simulink model "QuadcopterSimModel_INDI_simple_Atti"  (R2018b)
settings: Solver=ode23  StartTime=0.0  StopTime=1000  FixedStep=sample_time  RelTol=1e-4  EnableMultiTasking=on
undefined symbols (not defined in the file): alt_ground, atmosphere, DiscIntNeverNeededParam, envir, fm_atti, g, jystck, pacer, pos_ref, sigbuilder_block, wind
libraries: unit_conversions_lib x3, aerolibfltsims x2, fmCopterAttiRedIndi_lib x1, filters_lib x1, atmosphere_lib x1, quadcopter_lib x1, aerolibanimutils x1, simulink x1, flightgear_visualization_lib x1, axes_transformation_lib x1, joystick_lib x1
settings Model: Creator=Yannic  LastModifiedBy=yannic
settings SolverCC: ZeroCrossControl=DisableAll
settings DataIOCC: LimitDataPoints=on  ReturnWorkspaceOutputs=on
settings OptimizationCC: LifeSpan=inf
settings DebuggingCC: ReadBeforeWriteMsg=DisableAll  WriteAfterWriteMsg=DisableAll  WriteAfterReadMsg=DisableAll  MultiTaskDSMMsg=none  AllowSymbolicDim=off  LibraryContextMissingDiagnostic=none  SFUnexpectedBacktrackingDiag=warning  SFNoUnconditionalDefaultTransitionDiag=warning  SFExecutionAtInitializationDiag=none
settings ModelReferenceCC: UpdateModelReferenceTargets=IfOutOfDate  PropagateSignalLabelsOutOfModel=off
settings SFSimCC: SFSimEcho=off  SimUseLocalCustomCode=off
settings RTWCC: RTWUseLocalCustomCode=off
settings CodeAppCC: StateflowObjectComments=on
settings GRTTargetCC: TargetLangStandard=C89/C90 (ANSI)
settings ConfigComp: CovMetricSettings=dw  CovHtmlReporting=on  CovSaveCumulativeToWorkspaceVar=on  CovSaveSingleToWorkspaceVar=on  CovExternalEMLEnable=off

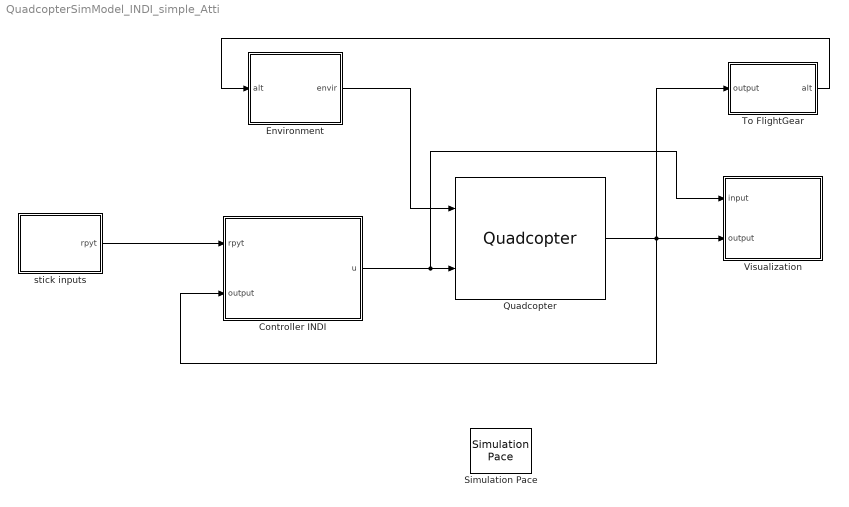
== system QuadcopterSimModel_INDI_simple_Atti ==
  Controller INDI : Subsystem
  Environment : Subsystem
  Quadcopter : quadcopter_lib/Quadcopter  copter_=copter  IC_=IC  grnd_=grnd
      settings: SourceProductName=LADAC
  Simulation Pace : aerolibanimutils/Simulation Pace  SimulationPace=pacer.pace  SleepMode=Auto  OutputPaceError=off  SampleTime=pacer.sample_time
  To FlightGear : Subsystem
  Visualization : Subsystem
  stick inputs : Subsystem
  wires:
  Environment/1(envir) -> Quadcopter/1
  stick inputs/1(rpyt) -> Controller INDI/1(rpyt)
  Quadcopter/1 -> To FlightGear/1(output), Visualization/2(output), Controller INDI/2(output)
  To FlightGear/1(alt) -> Environment/1(alt)
  Controller INDI/1(u) -> Quadcopter/2, Visualization/1(input)

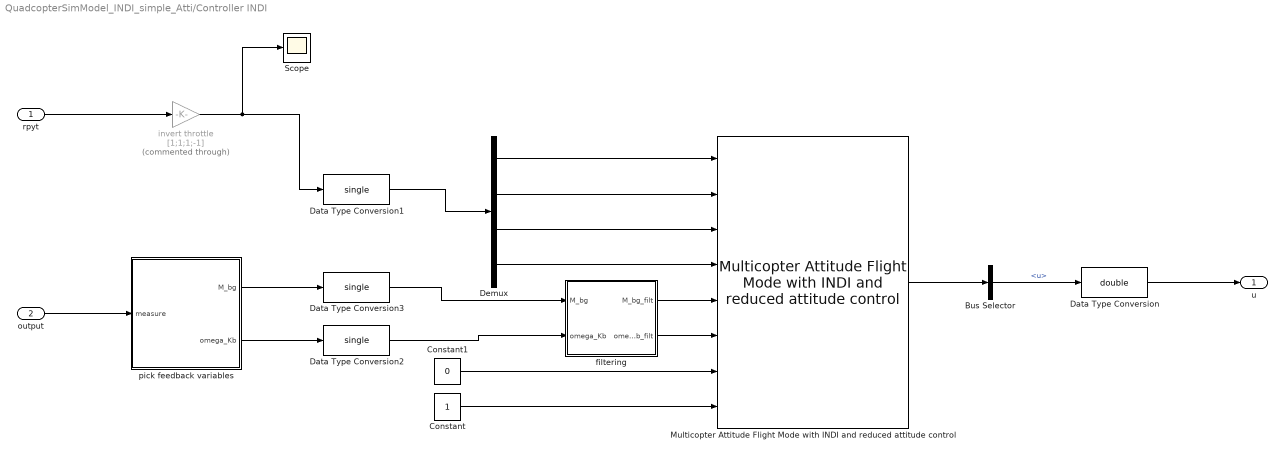
== system QuadcopterSimModel_INDI_simple_Atti/Controller INDI ==
  rpyt : Inport  OutDataTypeStr=double
  output : Inport  Port=2
  Bus Selector : BusSelector  OutputSignals=u
  Constant : Constant  OutDataTypeStr=Inherit: Inherit via back propagation
  Constant1 : Constant  Value=0  OutDataTypeStr=Inherit: Inherit via back propagation
  Data Type Conversion : DataTypeConversion  OutDataTypeStr=double
  Data Type Conversion1 : DataTypeConversion  OutDataTypeStr=single
  Data Type Conversion2 : DataTypeConversion  OutDataTypeStr=single
  Data Type Conversion3 : DataTypeConversion  OutDataTypeStr=single
  Demux : Demux
  Multicopter Attitude Flight Mode with INDI and reduced attitude control : fmCopterAttiRedIndi_lib/Multicopter Attitude Flight Mode with INDI and reduced attitude control  fm=fm_atti
  Scope : Scope
  filtering : Subsystem
  invert throttle : Gain  Commented=through  Gain=[1;1;1;-1]
  pick feedback variables : Subsystem
  u : Outport  OutDataTypeStr=double  PortDimensions=4  SampleTime=[0.0025000000000000001,0]
  wires:
  rpyt/1 -> invert throttle/1
  output/1 -> pick feedback variables/1(measure)
  invert throttle/1 -> Scope/1, Data Type Conversion1/1
  pick feedback variables/2(omega_Kb) -> Data Type Conversion2/1
  pick feedback variables/1(M_bg) -> Data Type Conversion3/1
  Multicopter Attitude Flight Mode with INDI and reduced attitude control/1 -> Bus Selector/1
  Data Type Conversion/1 -> u/1
  Data Type Conversion1/1 -> Demux/1
  Demux/4 -> Multicopter Attitude Flight Mode with INDI and reduced attitude control/4
  Demux/3 -> Multicopter Attitude Flight Mode with INDI and reduced attitude control/3
  Demux/2 -> Multicopter Attitude Flight Mode with INDI and reduced attitude control/2
  Demux/1 -> Multicopter Attitude Flight Mode with INDI and reduced attitude control/1
  Constant/1 -> Multicopter Attitude Flight Mode with INDI and reduced attitude control/8
  Constant1/1 -> Multicopter Attitude Flight Mode with INDI and reduced attitude control/7
  Bus Selector/1 -> Data Type Conversion/1  "<u>"
  Data Type Conversion3/1 -> filtering/1(M_bg)
  filtering/1(M_bg_filt) -> Multicopter Attitude Flight Mode with INDI and reduced attitude control/5
  filtering/2(omega_Kb_filt) -> Multicopter Attitude Flight Mode with INDI and reduced attitude control/6
  Data Type Conversion2/1 -> filtering/2(omega_Kb)

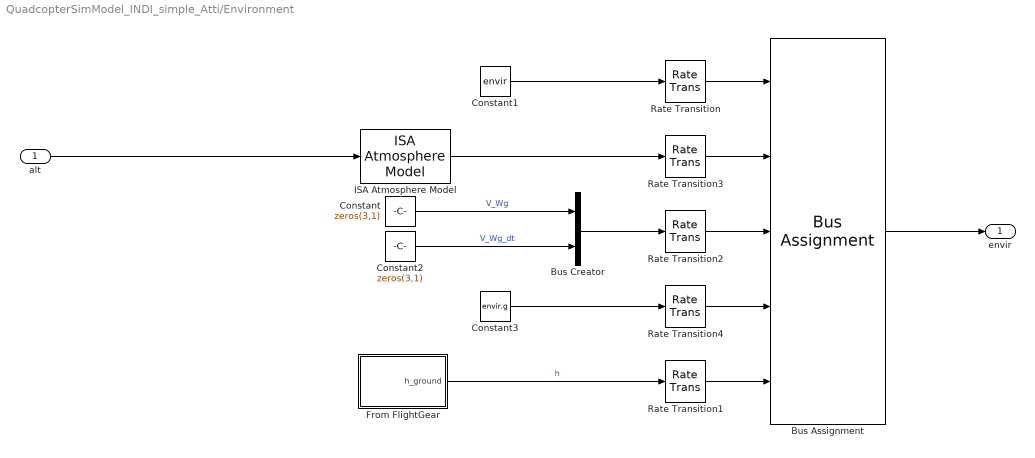
== system QuadcopterSimModel_INDI_simple_Atti/Environment ==
  alt : Inport
  Bus Assignment : BusAssignment  AssignedSignals=atmosphere,wind,g,alt_ground
  Bus Creator : BusCreator  Inputs=2
  Constant : Constant  Value=zeros(3,1)
  Constant1 : Constant  Value=envir  OutDataTypeStr=Bus: envirBus
  Constant2 : Constant  Value=zeros(3,1)
  Constant3 : Constant  Value=envir.g
  From FlightGear : Subsystem
  ISA Atmosphere Model : atmosphere_lib/ISA Atmosphere Model  SystemSampleTime=-1
      settings: SourceProductName=LADAC
  Rate Transition{,1..4} (5 alike) : RateTransition
  envir : Outport
  wires:
  From FlightGear/1(h_ground) -> Rate Transition1/1  "h"
  Rate Transition2/1 -> Bus Assignment/3
  Rate Transition3/1 -> Bus Assignment/2
  Bus Assignment/1 -> envir/1
  Rate Transition/1 -> Bus Assignment/1
  ISA Atmosphere Model/1 -> Rate Transition3/1
  Constant/1 -> Bus Creator/1  "V_Wg"
  Rate Transition1/1 -> Bus Assignment/5
  Constant1/1 -> Rate Transition/1
  alt/1 -> ISA Atmosphere Model/1
  Bus Creator/1 -> Rate Transition2/1
  Constant2/1 -> Bus Creator/2  "V_Wg_dt"
  Rate Transition4/1 -> Bus Assignment/4
  Constant3/1 -> Rate Transition4/1

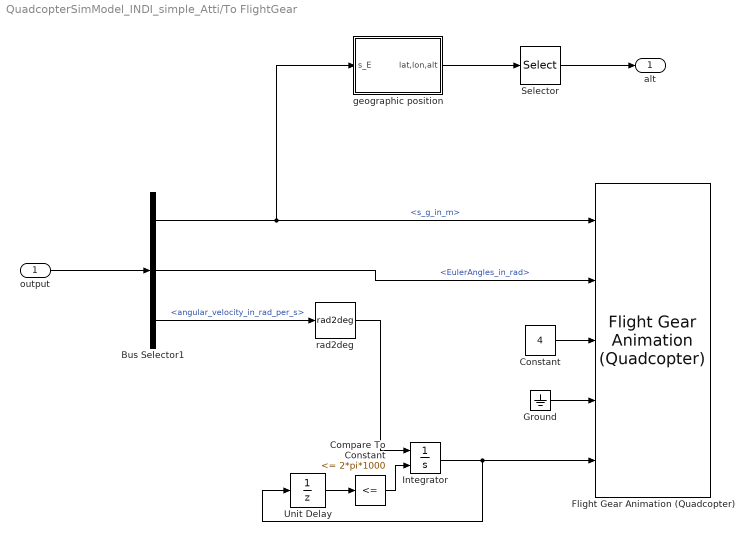
== system QuadcopterSimModel_INDI_simple_Atti/To FlightGear ==
  output : Inport
  Bus Selector1 : BusSelector  OutputSignals=rigidBodyBus.s_g_in_m,rigidBodyBus.EulerAngles_in_rad,motorBus.angular_velocity_in_rad_per_s
  Compare To Constant : simulink/Logic and Bit Operations/Compare To Constant  relop=<=  const=2*pi*1000  OutDataTypeStr=boolean
  Constant : Constant  Value=4
  Flight Gear Animation (Quadcopter) : flightgear_visualization_lib/Flight Gear Animation (Quadcopter)  inital_lat=pos_ref.lat  inital_long=pos_ref.lon  inital_height=pos_ref.alt  remoteURL=fg.remoteURL  remotePort=fg.remotePort
      settings: SourceProductName=LADAC
  Ground : Ground
  Integrator : Integrator  ExternalReset=rising
  Selector : Selector  InputPortWidth=3  IndexOptions=Index vector (dialog)  Indices=3  OutputSizes=1
  Unit Delay : UnitDelay  SampleTime=-1
  geographic position : Subsystem
  rad2deg : unit_conversions_lib/rad2deg
      settings: SourceProductName=LADAC
  alt : Outport
  wires:
  Bus Selector1/1 -> geographic position/1(s_E), Flight Gear Animation (Quadcopter)/1  "<s_g_in_m>"
  output/1 -> Bus Selector1/1
  geographic position/1(lat,lon,alt) -> Selector/1
  Bus Selector1/2 -> Flight Gear Animation (Quadcopter)/2  "<EulerAngles_in_rad>"
  Bus Selector1/3 -> rad2deg/1  "<angular_velocity_in_rad_per_s>"
  Selector/1 -> alt/1
  Constant/1 -> Flight Gear Animation (Quadcopter)/3
  Ground/1 -> Flight Gear Animation (Quadcopter)/4
  Integrator/1 -> Unit Delay/1, Flight Gear Animation (Quadcopter)/5
  Unit Delay/1 -> Compare To Constant/1
  Compare To Constant/1 -> Integrator/2
  rad2deg/1 -> Integrator/1

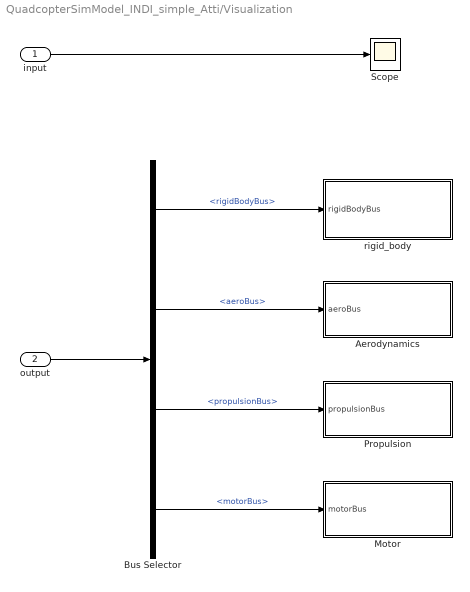
== system QuadcopterSimModel_INDI_simple_Atti/Visualization ==
  input : Inport
  output : Inport  Port=2
  Aerodynamics : Subsystem
  Bus Selector : BusSelector  OutputSignals=rigidBodyBus,aeroBus,propulsionBus,motorBus
  Motor : Subsystem
  Propulsion : Subsystem
  Scope : Scope
  rigid_body : Subsystem
  wires:
  output/1 -> Bus Selector/1
  Bus Selector/1 -> rigid_body/1(rigidBodyBus)  "<rigidBodyBus>"
  Bus Selector/2 -> Aerodynamics/1(aeroBus)  "<aeroBus>"
  Bus Selector/3 -> Propulsion/1(propulsionBus)  "<propulsionBus>"
  Bus Selector/4 -> Motor/1(motorBus)  "<motorBus>"
  input/1 -> Scope/1

== system QuadcopterSimModel_INDI_simple_Atti/stick inputs ==
  Calibrated Joystick : joystick_lib/Calibrated Joystick  jystck=jystck
      settings: SourceProductName=LADAC
  Constant1 : Constant  Value=jystck.enable
  Scope : Scope
  Selector2 : Selector  InputPortWidth=8  IndexOptions=Index vector (dialog)  Indices=[1,2,3,4]  OutputSizes=1
  Signal builder : Subsystem
  Switch1 : Switch  Criteria=u2 > Threshold
  rpyt : Outport
  wires:
  Switch1/1 -> Selector2/1, Scope/1
  Calibrated Joystick/1 -> Switch1/1
  Constant1/1 -> Calibrated Joystick/Enable, Switch1/2
  Signal builder/1(r) -> Switch1/3
  Selector2/1 -> rpyt/1

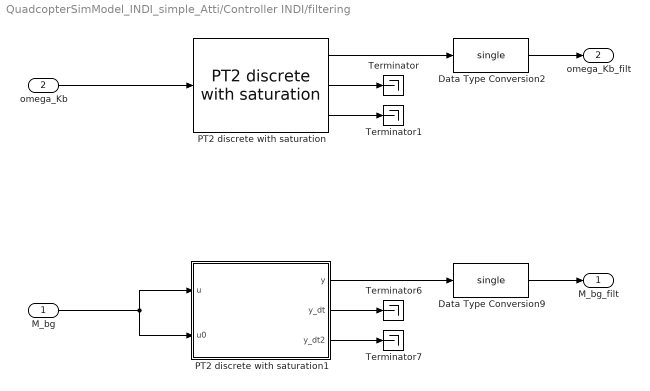
== system QuadcopterSimModel_INDI_simple_Atti/Controller INDI/filtering ==
  M_bg : Inport
  omega_Kb : Inport  Port=2
  Data Type Conversion2 : DataTypeConversion  OutDataTypeStr=single
  Data Type Conversion9 : DataTypeConversion  OutDataTypeStr=single
  PT2 discrete with saturation : filters_lib/PT2 discrete with saturation  omega=fm_atti.sens_filt.omega  d=fm_atti.sens_filt.D  x_dt2_max=inf  x_dt2_min=-inf  x_dt_max=inf  x_dt_min=-inf  x_max=inf  x_min=-inf  x_init=0  x_dt_init=0
      settings: SourceProductName=LADAC
  PT2 discrete with saturation1 : Subsystem  mask{omega=fm_atti.sens_filt.omega, d=fm_atti.sens_filt.D, x_dt2_max=inf, x_dt2_min=-inf, x_dt_max=inf, x_dt_min=-inf, x_max=inf, x_min=-inf, x_init=0, x_dt_init=0}
      mask prompts: omega "Natural frequency"; d "Damping ratio"; x_dt2_max "Maximum acceleration"; x_dt2_min "Minimum acceleration"; x_dt_max "Maximum rate"; x_dt_min "Minimum rate"; x_max "Maximum position"; x_min "Minimum position"; x_init "Initial position"; x_dt_init "Initial rate"
  Terminator{,1,6..7} (4 alike) : Terminator
  M_bg_filt : Outport
  omega_Kb_filt : Outport  Port=2
  wires:
  omega_Kb/1 -> PT2 discrete with saturation/1
  PT2 discrete with saturation/1 -> Data Type Conversion2/1
  M_bg/1 -> PT2 discrete with saturation1/2(u0), PT2 discrete with saturation1/1(u)
  PT2 discrete with saturation1/1(y) -> Data Type Conversion9/1
  PT2 discrete with saturation/2 -> Terminator/1
  PT2 discrete with saturation/3 -> Terminator1/1
  PT2 discrete with saturation1/2(y_dt) -> Terminator6/1
  PT2 discrete with saturation1/3(y_dt2) -> Terminator7/1
  Data Type Conversion9/1 -> M_bg_filt/1
  Data Type Conversion2/1 -> omega_Kb_filt/1

== system QuadcopterSimModel_INDI_simple_Atti/Controller INDI/pick feedback variables ==
  measure : Inport
  Bus Selector1 : BusSelector  OutputSignals=rigidBodyBus.omega_Kb_in_rad_per_s,rigidBodyBus.M_bg_in_1
  M_bg : Outport
  omega_Kb : Outport  Port=2
  wires:
  measure/1 -> Bus Selector1/1
  Bus Selector1/2 -> M_bg/1  "<M_bg_in_1>"
  Bus Selector1/1 -> omega_Kb/1  "<omega_Kb_in_rad_per_s>"

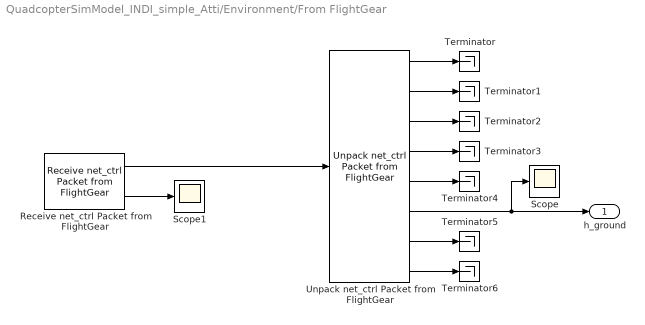
== system QuadcopterSimModel_INDI_simple_Atti/Environment/From FlightGear ==
  Receive net_ctrl Packet from FlightGear : aerolibfltsims/Receive net_ctrl Packet from FlightGear  FlightGearVersion=v3.4  ReceiveAddress=127.0.0.1  ReceivePort=5503  ReceiveWidth=744  varLen=off  SampleTime=1/5  packetFlag=on
      settings: AttributesFormatString=Version Selected:\n%<FlightGearVersion>  SourceProductName=Aerospace Blockset  SourceProductBaseCode=AE
  Scope : Scope
  Scope1 : Scope
  Terminator{,1..6} (7 alike) : Terminator
  Unpack net_ctrl Packet from FlightGear : aerolibfltsims/Unpack net_ctrl Packet from FlightGear  FlightGearVersion=v3.4  ShowControlSurfacePositionOutputs=off  ShowEngineFuelOutputs=off  ShowLandingGearOutputs=off  ShowAvionicOutputs=off  ShowEnvironmentOutputs=on  SampleTime=1/5  packetVersion=27
      settings: AttributesFormatString=Version Selected: %<FlightGearVersion>  SourceProductName=Aerospace Blockset  SourceProductBaseCode=AE
  h_ground : Outport
  wires:
  Unpack net_ctrl Packet from FlightGear/4 -> Terminator3/1
  Unpack net_ctrl Packet from FlightGear/5 -> Terminator4/1
  Receive net_ctrl Packet from FlightGear/1 -> Unpack net_ctrl Packet from FlightGear/1
  Unpack net_ctrl Packet from FlightGear/2 -> Terminator1/1
  Unpack net_ctrl Packet from FlightGear/7 -> Terminator5/1
  Unpack net_ctrl Packet from FlightGear/1 -> Terminator/1
  Unpack net_ctrl Packet from FlightGear/3 -> Terminator2/1
  Unpack net_ctrl Packet from FlightGear/8 -> Terminator6/1
  Unpack net_ctrl Packet from FlightGear/6 -> Scope/1, h_ground/1
  Receive net_ctrl Packet from FlightGear/2 -> Scope1/1

== system QuadcopterSimModel_INDI_simple_Atti/To FlightGear/geographic position ==
  s_E : Inport
  Constant : Constant  Value=pos_ref.lat
  Constant1 : Constant  Value=pos_ref.lon
  Constant2 : Constant  Value=pos_ref.alt
  Mux : Mux  Inputs=3
  Scope : Scope  NumInputPorts=3
  "flat earth to lat, lon, alt" : axes_transformation_lib/NED to lat, lon, alt  SystemSampleTime=-1
      settings: SourceProductName=LADAC
  lat,lon,alt : Outport
  wires:
  Constant2/1 -> "flat earth to lat, lon, alt"/3
  Constant1/1 -> "flat earth to lat, lon, alt"/2
  "flat earth to lat, lon, alt"/3 -> Scope/3, Mux/3
  Constant/1 -> "flat earth to lat, lon, alt"/1
  Mux/1 -> lat,lon,alt/1
  s_E/1 -> "flat earth to lat, lon, alt"/4
  "flat earth to lat, lon, alt"/2 -> Mux/2, Scope/2
  "flat earth to lat, lon, alt"/1 -> Mux/1, Scope/1

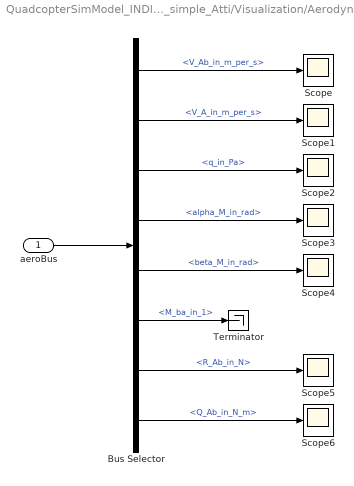
== system QuadcopterSimModel_INDI_simple_Atti/Visualization/Aerodynamics ==
  aeroBus : Inport
  Bus Selector : BusSelector  OutputSignals=V_Ab_in_m_per_s,V_A_in_m_per_s,q_in_Pa,angles.alpha_M_in_rad,angles.beta_M_in_rad,M_ba_in_1,R_Ab_in_N,Q_Ab_in_N_m
  Scope{,1..6} (7 alike) : Scope
  Terminator : Terminator
  wires:
  aeroBus/1 -> Bus Selector/1
  Bus Selector/1 -> Scope/1  "<V_Ab_in_m_per_s>"
  Bus Selector/2 -> Scope1/1  "<V_A_in_m_per_s>"
  Bus Selector/3 -> Scope2/1  "<q_in_Pa>"
  Bus Selector/4 -> Scope3/1  "<alpha_M_in_rad>"
  Bus Selector/5 -> Scope4/1  "<beta_M_in_rad>"
  Bus Selector/6 -> Terminator/1  "<M_ba_in_1>"
  Bus Selector/7 -> Scope5/1  "<R_Ab_in_N>"
  Bus Selector/8 -> Scope6/1  "<Q_Ab_in_N_m>"

== system QuadcopterSimModel_INDI_simple_Atti/Visualization/Motor ==
  motorBus : Inport
  Bus Selector : BusSelector  OutputSignals=angular_acceleration_in_rad_per_square_s,angular_velocity_in_rad_per_s
  Scope : Scope
  Scope1 : Scope
  wires:
  Bus Selector/1 -> Scope/1  "<angular_acceleration_in_rad_per_square_s>"
  motorBus/1 -> Bus Selector/1
  Bus Selector/2 -> Scope1/1  "<angular_velocity_in_rad_per_s>"

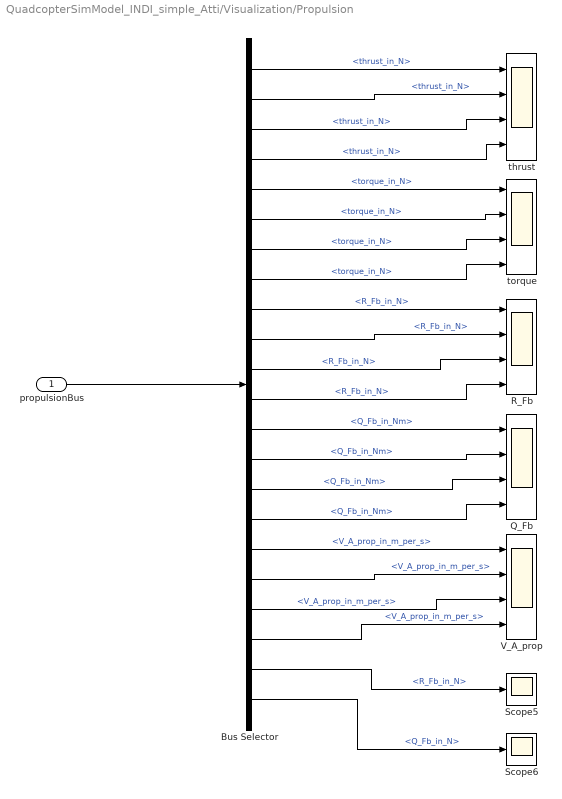
== system QuadcopterSimModel_INDI_simple_Atti/Visualization/Propulsion ==
  propulsionBus : Inport
  Bus Selector : BusSelector  OutputSignals=propeller_1.thrust_in_N,propeller_2.thrust_in_N,propeller_3.thrust_in_N,propeller_4.thrust_in_N,propeller_1.torque_in_N,propeller_2.torque_in_N,propeller_3.torque_in_N,propeller_4.torque_in_N,propeller_1.R_Fb_in_N,propeller_2.R_Fb_in_N,propeller_3.R_Fb_in_N,propeller_4.R_Fb_in_N,propeller_1.Q_Fb_in_Nm,propeller_2.Q_Fb_in_Nm,propeller_3.Q_Fb_in_Nm,propeller_4.Q_Fb_in_Nm,propeller_1.V_A_prop_in_m_per_s,propeller_2.V_A_prop_in_m_per_s,propeller_3.V_A_prop_in_m_per_s,propeller_4.V_A_prop_in_m_per_s,R_Fb_in_N,Q_Fb_in_N
  Q_Fb : Scope  NumInputPorts=4
  R_Fb : Scope  NumInputPorts=4
  Scope5 : Scope
  Scope6 : Scope
  V_A_prop : Scope  NumInputPorts=4
  thrust : Scope  NumInputPorts=4
  torque : Scope  NumInputPorts=4
  wires:
  propulsionBus/1 -> Bus Selector/1
  Bus Selector/1 -> thrust/1  "<thrust_in_N>"
  Bus Selector/2 -> thrust/2  "<thrust_in_N>"
  Bus Selector/3 -> thrust/3  "<thrust_in_N>"
  Bus Selector/4 -> thrust/4  "<thrust_in_N>"
  Bus Selector/5 -> torque/1  "<torque_in_N>"
  Bus Selector/6 -> torque/2  "<torque_in_N>"
  Bus Selector/7 -> torque/3  "<torque_in_N>"
  Bus Selector/8 -> torque/4  "<torque_in_N>"
  Bus Selector/9 -> R_Fb/1  "<R_Fb_in_N>"
  Bus Selector/10 -> R_Fb/2  "<R_Fb_in_N>"
  Bus Selector/11 -> R_Fb/3  "<R_Fb_in_N>"
  Bus Selector/12 -> R_Fb/4  "<R_Fb_in_N>"
  Bus Selector/13 -> Q_Fb/1  "<Q_Fb_in_Nm>"
  Bus Selector/14 -> Q_Fb/2  "<Q_Fb_in_Nm>"
  Bus Selector/15 -> Q_Fb/3  "<Q_Fb_in_Nm>"
  Bus Selector/16 -> Q_Fb/4  "<Q_Fb_in_Nm>"
  Bus Selector/17 -> V_A_prop/1  "<V_A_prop_in_m_per_s>"
  Bus Selector/18 -> V_A_prop/2  "<V_A_prop_in_m_per_s>"
  Bus Selector/19 -> V_A_prop/3  "<V_A_prop_in_m_per_s>"
  Bus Selector/20 -> V_A_prop/4  "<V_A_prop_in_m_per_s>"
  Bus Selector/21 -> Scope5/1  "<R_Fb_in_N>"
  Bus Selector/22 -> Scope6/1  "<Q_Fb_in_N>"

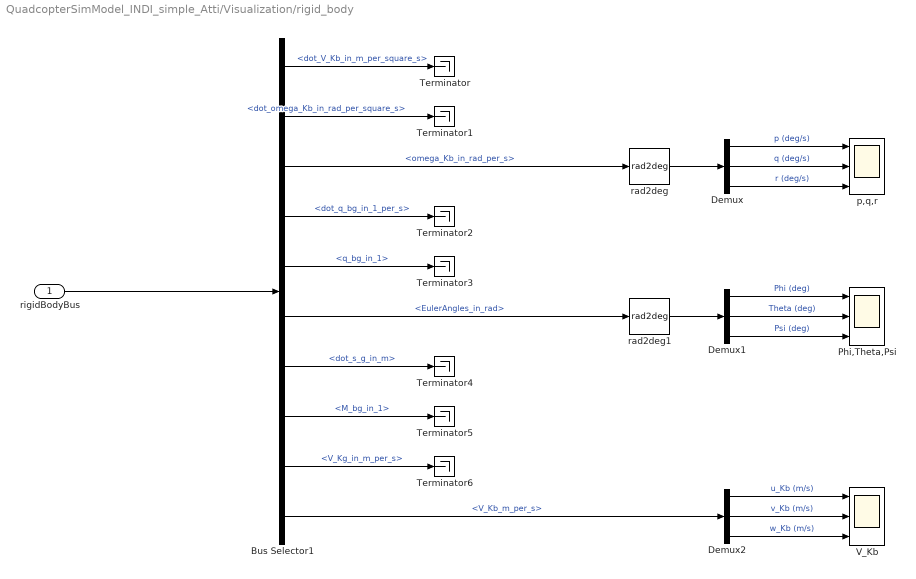
== system QuadcopterSimModel_INDI_simple_Atti/Visualization/rigid_body ==
  rigidBodyBus : Inport
  Bus Selector1 : BusSelector  OutputSignals=dot_V_Kb_in_m_per_square_s,dot_omega_Kb_in_rad_per_square_s,omega_Kb_in_rad_per_s,dot_q_bg_in_1_per_s,q_bg_in_1,EulerAngles_in_rad,dot_s_g_in_m,M_bg_in_1,V_Kg_in_m_per_s,V_Kb_m_per_s
  Demux : Demux  Outputs=3
  Demux1 : Demux  Outputs=3
  Demux2 : Demux  Outputs=3
  Phi,Theta,Psi : Scope  NumInputPorts=3
  Terminator{,1..6} (7 alike) : Terminator
  V_Kb : Scope  NumInputPorts=3
  p,q,r : Scope  NumInputPorts=3
  rad2deg : unit_conversions_lib/rad2deg
      settings: SourceProductName=LADAC
  rad2deg1 : unit_conversions_lib/rad2deg
      settings: SourceProductName=LADAC
  wires:
  Demux/1 -> p,q,r/1  "p (deg/s)"
  Demux1/2 -> Phi,Theta,Psi/2  "Theta (deg)"
  rad2deg/1 -> Demux/1
  Demux1/1 -> Phi,Theta,Psi/1  "Phi (deg)"
  Demux1/3 -> Phi,Theta,Psi/3  "Psi (deg)"
  Demux2/3 -> V_Kb/3  "w_Kb (m/s)"
  Bus Selector1/7 -> Terminator4/1  "<dot_s_g_in_m>"
  Bus Selector1/6 -> rad2deg1/1  "<EulerAngles_in_rad>"
  Bus Selector1/3 -> rad2deg/1  "<omega_Kb_in_rad_per_s>"
  Demux/3 -> p,q,r/3  "r (deg/s)"
  Bus Selector1/1 -> Terminator/1  "<dot_V_Kb_in_m_per_square_s>"
  Demux2/2 -> V_Kb/2  "v_Kb (m/s)"
  Demux/2 -> p,q,r/2  "q (deg/s)"
  rad2deg1/1 -> Demux1/1
  Bus Selector1/5 -> Terminator3/1  "<q_bg_in_1>"
  Demux2/1 -> V_Kb/1  "u_Kb (m/s)"
  Bus Selector1/10 -> Demux2/1  "<V_Kb_m_per_s>"
  rigidBodyBus/1 -> Bus Selector1/1
  Bus Selector1/8 -> Terminator5/1  "<M_bg_in_1>"
  Bus Selector1/4 -> Terminator2/1  "<dot_q_bg_in_1_per_s>"
  Bus Selector1/2 -> Terminator1/1  "<dot_omega_Kb_in_rad_per_square_s>"
  Bus Selector1/9 -> Terminator6/1  "<V_Kg_in_m_per_s>"

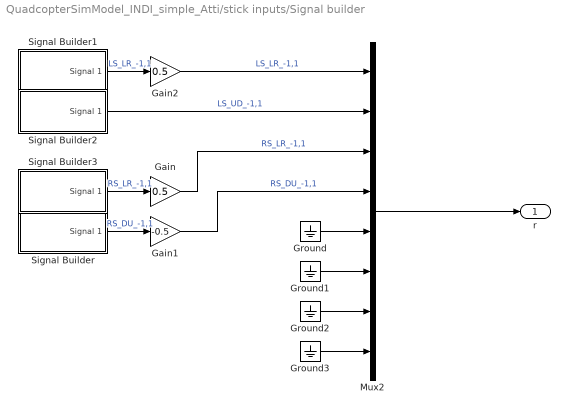
== system QuadcopterSimModel_INDI_simple_Atti/stick inputs/Signal builder ==
  Gain : Gain  Gain=0.5
  Gain1 : Gain  Gain=-0.5
  Gain2 : Gain  Gain=0.5
  Ground{,1..3} (4 alike) : Ground
  Mux2 : Mux  Inputs=8
  Signal Builder : Subsystem  Tag=STV Subsys  LoadFcn=sigbuilder_block('load');  StartFcn=sigbuilder_block('start');  StopFcn=sigbuilder_block('stop');  ClipboardFcn=sigbuilder_block('clipboard');  mask(Sigbuilder block){tuvar=[0:10]}
      mask help: Simulink:masks:SigbuilderBlock_MD
      mask init:
      | if ~strcmp(get_param(bdroot(gcbh),'SimulationStatus'),'stopped') tuvar = sigbuilder_block('maskInit'); end
      settings: CopyFcn=sigbuilder_block('copy');  DeleteFcn=sigbuilder_block('delete');  ModelCloseFcn=sigbuilder_block('modelClose');  PreSaveFcn=sigbuilder_block('preSave');  PauseFcn=sigbuilder_block('pause');  ContinueFcn=sigbuilder_block('continue');  NameChangeFcn=sigbuilder_block('namechange');  OpenFcn=sigbuilder_block('open',[426 42.75 821.25 509.25 ]);  CloseFcn=sigbuilder_block('close');
      mask Display: plot(0, 0, 100, 100,[2, 2, 32, 32, 2], [68, 8, 8, 68, 68],[32, 2], [38, 38], [32, 19, 2],[53, 60, 44], [32, 17, 17, 2],[16, 16, 31, 31]);txt = getActiveGroup(gcbh);text(2, 100, txt,'verticalAlignment', 'top');
  Signal Builder1 : Subsystem  Tag=STV Subsys  LoadFcn=sigbuilder_block('load');  StartFcn=sigbuilder_block('start');  StopFcn=sigbuilder_block('stop');  ClipboardFcn=sigbuilder_block('clipboard');  mask(Sigbuilder block){tuvar=[0:10]}
      mask help: Simulink:masks:SigbuilderBlock_MD
      mask init:
      | if ~strcmp(get_param(bdroot(gcbh),'SimulationStatus'),'stopped') tuvar = sigbuilder_block('maskInit'); end
      settings: CopyFcn=sigbuilder_block('copy');  DeleteFcn=sigbuilder_block('delete');  ModelCloseFcn=sigbuilder_block('modelClose');  PreSaveFcn=sigbuilder_block('preSave');  PauseFcn=sigbuilder_block('pause');  ContinueFcn=sigbuilder_block('continue');  NameChangeFcn=sigbuilder_block('namechange');  OpenFcn=sigbuilder_block('open',[429.75 123 565.5 444.75 ]);  CloseFcn=sigbuilder_block('close');
      mask Display: plot(0, 0, 100, 100,[2, 2, 32, 32, 2], [68, 8, 8, 68, 68],[32, 2], [38, 38], [32, 19, 2],[53, 60, 44], [32, 17, 17, 2],[16, 16, 31, 31]);txt = getActiveGroup(gcbh);text(2, 100, txt,'verticalAlignment', 'top');
  Signal Builder2 : Subsystem  Tag=STV Subsys  LoadFcn=sigbuilder_block('load');  StartFcn=sigbuilder_block('start');  StopFcn=sigbuilder_block('stop');  ClipboardFcn=sigbuilder_block('clipboard');  mask(Sigbuilder block){tuvar=[0:10]}
      mask help: Simulink:masks:SigbuilderBlock_MD
      mask init:
      | if ~strcmp(get_param(bdroot(gcbh),'SimulationStatus'),'stopped') tuvar = sigbuilder_block('maskInit'); end
      settings: CopyFcn=sigbuilder_block('copy');  DeleteFcn=sigbuilder_block('delete');  ModelCloseFcn=sigbuilder_block('modelClose');  PreSaveFcn=sigbuilder_block('preSave');  PauseFcn=sigbuilder_block('pause');  ContinueFcn=sigbuilder_block('continue');  NameChangeFcn=sigbuilder_block('namechange');  OpenFcn=sigbuilder_block('open',[411 0 603 557.25 ]);  CloseFcn=sigbuilder_block('close');
      mask Display: plot(0, 0, 100, 100,[2, 2, 32, 32, 2], [68, 8, 8, 68, 68],[32, 2], [38, 38], [32, 19, 2],[53, 60, 44], [32, 17, 17, 2],[16, 16, 31, 31]);txt = getActiveGroup(gcbh);text(2, 100, txt,'verticalAlignment', 'top');
  Signal Builder3 : Subsystem  Tag=STV Subsys  LoadFcn=sigbuilder_block('load');  StartFcn=sigbuilder_block('start');  StopFcn=sigbuilder_block('stop');  ClipboardFcn=sigbuilder_block('clipboard');  mask(Sigbuilder block){tuvar=[0:10]}
      mask help: Simulink:masks:SigbuilderBlock_MD
      mask init:
      | if ~strcmp(get_param(bdroot(gcbh),'SimulationStatus'),'stopped') tuvar = sigbuilder_block('maskInit'); end
      settings: CopyFcn=sigbuilder_block('copy');  DeleteFcn=sigbuilder_block('delete');  ModelCloseFcn=sigbuilder_block('modelClose');  PreSaveFcn=sigbuilder_block('preSave');  PauseFcn=sigbuilder_block('pause');  ContinueFcn=sigbuilder_block('continue');  NameChangeFcn=sigbuilder_block('namechange');  OpenFcn=sigbuilder_block('open',[433.5 161.25 558 422.25 ]);  CloseFcn=sigbuilder_block('close');
      mask Display: plot(0, 0, 100, 100,[2, 2, 32, 32, 2], [68, 8, 8, 68, 68],[32, 2], [38, 38], [32, 19, 2],[53, 60, 44], [32, 17, 17, 2],[16, 16, 31, 31]);txt = getActiveGroup(gcbh);text(2, 100, txt,'verticalAlignment', 'top');
  r : Outport
  wires:
  Ground3/1 -> Mux2/8
  Gain2/1 -> Mux2/1  "LS_LR_-1,1"
  Ground1/1 -> Mux2/6
  Ground2/1 -> Mux2/7
  Mux2/1 -> r/1
  Signal Builder2/1(Signal 1) -> Mux2/2  "LS_UD_-1,1"
  Gain/1 -> Mux2/3  "RS_LR_-1,1"
  Ground/1 -> Mux2/5
  Gain1/1 -> Mux2/4  "RS_DU_-1,1"
  Signal Builder3/1(Signal 1) -> Gain/1  "RS_LR_-1,1"
  Signal Builder/1(Signal 1) -> Gain1/1  "RS_DU_-1,1"
  Signal Builder1/1(Signal 1) -> Gain2/1  "LS_LR_-1,1"

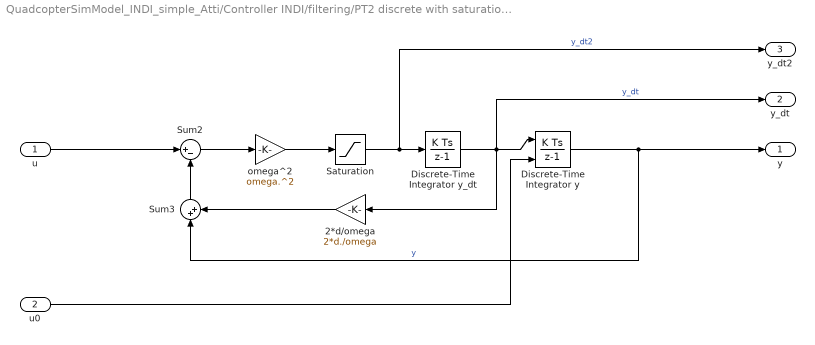
== system QuadcopterSimModel_INDI_simple_Atti/Controller INDI/filtering/PT2 discrete with saturation1 ==
  u : Inport
  u0 : Inport  Port=2
  2*d/omega : Gain  Gain=2*d./omega
  Discrete-Time Integrator y : DiscreteIntegrator  InitialConditionSource=external  InitialCondition=x_init  SampleTime=-1  OutDataTypeStr=Inherit: Inherit via back propagation  LimitOutput=on  UpperSaturationLimit=x_max  LowerSaturationLimit=x_min  ICPrevOutput=DiscIntNeverNeededParam  ICPrevScaledInput=DiscIntNeverNeededParam
  Discrete-Time Integrator y_dt : DiscreteIntegrator  InitialCondition=x_dt_init  SampleTime=-1  OutDataTypeStr=Inherit: Inherit via back propagation  LimitOutput=on  UpperSaturationLimit=x_dt_max  LowerSaturationLimit=x_dt_min  ICPrevOutput=DiscIntNeverNeededParam  ICPrevScaledInput=DiscIntNeverNeededParam
  Saturation : Saturate  UpperLimit=x_dt2_max  LowerLimit=x_dt2_min
  Sum2 : Sum  Inputs=|+-
  Sum3 : Sum  Inputs=|++
  omega^2 : Gain  Gain=omega.^2
  y : Outport
  y_dt : Outport  Port=2
  y_dt2 : Outport  Port=3
  wires:
  Saturation/1 -> y_dt2/1, Discrete-Time Integrator y_dt/1  "y_dt2"
  omega^2/1 -> Saturation/1
  Sum3/1 -> Sum2/2
  u/1 -> Sum2/1
  2*d/omega/1 -> Sum3/2
  Sum2/1 -> omega^2/1
  Discrete-Time Integrator y/1 -> Sum3/1, y/1  "y"
  Discrete-Time Integrator y_dt/1 -> 2*d/omega/1, y_dt/1, Discrete-Time Integrator y/1  "y_dt"
  u0/1 -> Discrete-Time Integrator y/2

== system QuadcopterSimModel_INDI_simple_Atti/stick inputs/Signal builder/Signal Builder ==
  Demux : Demux  Tag=STV Demux  Outputs=1
  FromWs : FromWorkspace  Tag=STV FromWs  VariableName=tuvar  SampleTime=0
      SigBuilderData=|
      | common.afterFinalStr = 'Extrapolate'
      | common.sampleTime = 0
      | dataSet.timeRange = [0 10]
      | dataSet.name = 'Group 1'
      | sbobj.Groups.Name = 'Group 1'
      | sbobj.Groups.Signals.Name = 'Signal 1'
      | sbobj.Groups.Signals.XData = [0 8 8 9.9 9.9 9.92 9.92 9.96 9.96 10]
      | sbobj.Groups.Signals.YData = [0 0 1 1 1.005 0.803 0.8 0.4 0 0]
  Signal 1 : Outport  Tag=STV Outport
  wires:
  Demux/1 -> Signal 1/1
  FromWs/1 -> Demux/1

== system QuadcopterSimModel_INDI_simple_Atti/stick inputs/Signal builder/Signal Builder1 ==
  Demux : Demux  Tag=STV Demux  Outputs=1
  FromWs : FromWorkspace  Tag=STV FromWs  VariableName=tuvar  SampleTime=0
      SigBuilderData=|
      | common.afterFinalStr = 'Extrapolate'
      | common.sampleTime = 0
      | dataSet.timeRange = [0 10]
      | dataSet.name = 'Group 1'
      | sbobj.Groups.Name = 'Group 1'
      | sbobj.Groups.Signals.Name = 'Signal 1'
      | sbobj.Groups.Signals.XData = [0 4 4 6 6 10]
      | sbobj.Groups.Signals.YData = [0 0 1 1 0 0]
  Signal 1 : Outport  Tag=STV Outport
  wires:
  Demux/1 -> Signal 1/1
  FromWs/1 -> Demux/1

== system QuadcopterSimModel_INDI_simple_Atti/stick inputs/Signal builder/Signal Builder2 ==
  Demux : Demux  Tag=STV Demux  Outputs=1
  FromWs : FromWorkspace  Tag=STV FromWs  VariableName=tuvar  SampleTime=0
      SigBuilderData=|
      | common.afterFinalStr = 'Extrapolate'
      | common.sampleTime = 0
      | dataSet.timeRange = [0 10]
      | dataSet.name = 'Group 1'
      | sbobj.Groups.Name = 'Group 1'
      | sbobj.Groups.Signals.Name = 'Signal 1'
      | sbobj.Groups.Signals.XData = [0 2 2 6 8 10]
      | sbobj.Groups.Signals.YData = [0 0 -1 -1 0 0]
  Signal 1 : Outport  Tag=STV Outport
  wires:
  FromWs/1 -> Demux/1
  Demux/1 -> Signal 1/1

== system QuadcopterSimModel_INDI_simple_Atti/stick inputs/Signal builder/Signal Builder3 ==
  Demux : Demux  Tag=STV Demux  Outputs=1
  FromWs : FromWorkspace  Tag=STV FromWs  VariableName=tuvar  SampleTime=0
      SigBuilderData=|
      | common.afterFinalStr = 'Extrapolate'
      | common.sampleTime = 0
      | dataSet.timeRange = [0 10]
      | dataSet.name = 'Group 1'
      | sbobj.Groups.Name = 'Group 1'
      | sbobj.Groups.Signals.Name = 'Signal 1'
      | sbobj.Groups.Signals.XData = [0 6 6 8 8 10]
      | sbobj.Groups.Signals.YData = [0 0 1 1 0 0]
  Signal 1 : Outport  Tag=STV Outport
  wires:
  Demux/1 -> Signal 1/1
  FromWs/1 -> Demux/1
